simulink model "Parents Phone-MS"  (R2023a)
settings: Solver=FixedStepAuto  StartTime=0.0  StopTime=inf  RelTol=1e-3
undefined symbols (not defined in the file): alti, latitude_, Longit, udp_recieve0x2810x29
libraries: androidcommunicationlib x5, androiduilib x3, androidaudiovideolib x1
settings Model: Creator=91942  LastModifiedBy=ketha
settings OptimizationCC: EnhancedBackFolding=on  PassReuseOutputArgsAs=Individual arguments  ZeroExternalMemoryAtStartup=off  ZeroInternalMemoryAtStartup=off  MaxStackSize=64  OptimizeBlockOrder=speed  DifferentSizesBufferReuse=on  OptimizationCustomize=off  EfficientTunableParamExpr=on
settings DebuggingCC: ParameterTunabilityLossMsg=error
settings HardwareCC: ProdBitPerLong=64  ProdLargestAtomicInteger=LongLong  ProdLargestAtomicFloat=Double  ProdLongLongMode=on  ProdHWDeviceType=ARM Compatible->ARM 64-bit (LP64)  UseEmbeddedCoderFeatures=off
settings SFSimCC: MATLABDynamicMemAlloc=off
settings RTWCC: Description=Embedded Coder  SystemTargetFile=ert.tlc  HardwareBoard=Android Device (64bit)  TLCOptions="-aInlineSetEventsForThisBaseRateFcn=TLC_FALSE -aSuppressMultiTaskScheduler=TLC_FALSE  -aRateBasedStepFcn=0"  TemplateMakefile=ert_default_tmf  RTWVerbose=off  Toolchain=Android SDK/NDK Tools
settings CodeAppCC: ForceParamTrailComments=on  IgnoreCustomStorageClasses=off  OperatorAnnotations=on  SimulinkDataObjDesc=on  SFDataObjDesc=on  InsertBlockDesc=on
settings ERTTargetCC: SupportNonInlinedSFcns=on

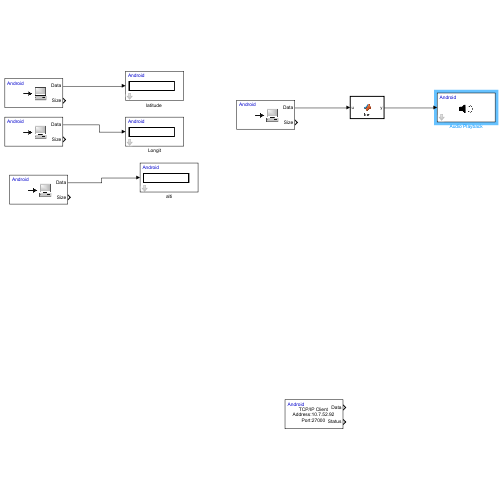
[thumbnail: Simulink's stored preview of the top-level diagram]
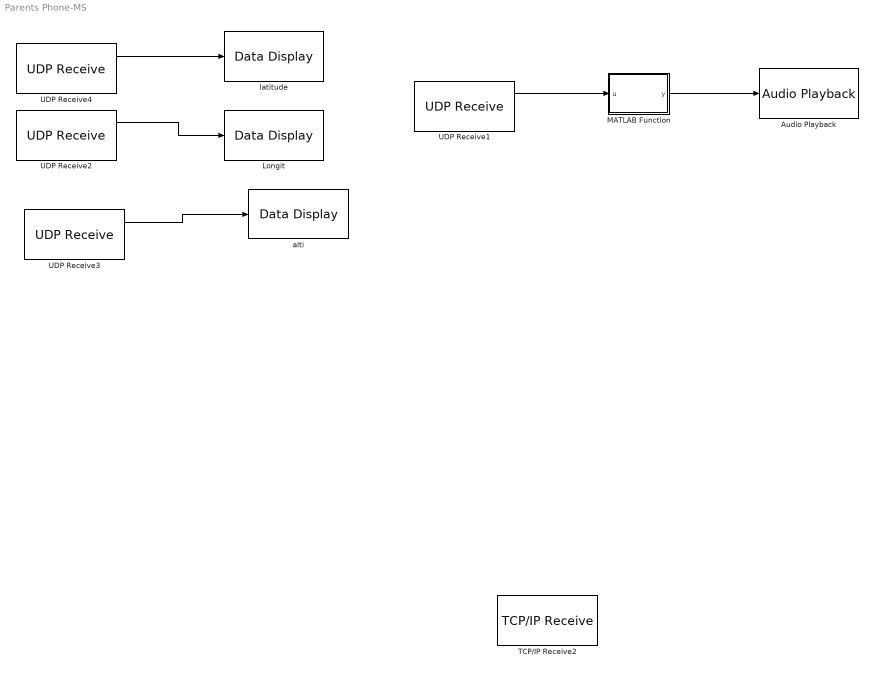
== system Parents Phone-MS ==
  Audio Playback : androidaudiovideolib/Audio Playback  SampleFreq=44100  AudioSamplingFreq=44100  SampleTime=0.1  DeviceStr=0  QueueDuration=0  BlockPlatform=Android
  Longit : androiduilib/Data Display  DataDisplayId=udp_recieve0x2810x29/Longit  Format=Float  Precision=6  SimulateUsing=Code generation  blockPlatform=Android
  MATLAB Function : MATLAB Function  TreatAsAtomicUnit=on
  TCP/IP Receive2 : androidcommunicationlib/TCP//IP Receive  TCPReceiveId=udp_recieve0x2810x29/TCP//IP_Receive2  Mode_=Client  LocalServerPort_=27000  RemoteAddr_=10.7.52.92  RemoteServerPort_=27000  DataType_=uint8  DataSize_=1  SampleTime_=0.1  ClientPortBindingSelection_=off  ClientPortToBind_=35000  BlockingMode_=off  BlockTimeout_=0.1
  UDP Receive1 : androidcommunicationlib/UDP Receive  localURL='0.0.0.0'  localPort=32000  remoteURL='0.0.0.0'  remotePort=-1  recvBufferSize=8192  signalDatatype=int16  dims=8820  isVarSize=off  showBlockingTime=off  blockingTime=0  sampletime=0.1  blockPlatform=Android
  UDP Receive2 : androidcommunicationlib/UDP Receive  localURL='0.0.0.0'  localPort=26000  remoteURL='0.0.0.0'  remotePort=-1  recvBufferSize=8192  signalDatatype=double  dims=1  isVarSize=off  showBlockingTime=off  blockingTime=0  sampletime=0.1  blockPlatform=Android
  UDP Receive3 : androidcommunicationlib/UDP Receive  localURL='0.0.0.0'  localPort=27000  remoteURL='0.0.0.0'  remotePort=-1  recvBufferSize=8192  signalDatatype=double  dims=1  isVarSize=off  showBlockingTime=off  blockingTime=0  sampletime=0.1  blockPlatform=Android
  UDP Receive4 : androidcommunicationlib/UDP Receive  localURL='0.0.0.0'  localPort=25000  remoteURL='0.0.0.0'  remotePort=-1  recvBufferSize=8192  signalDatatype=double  dims=1  isVarSize=off  showBlockingTime=off  blockingTime=0  sampletime=0.1  blockPlatform=Android
  alti : androiduilib/Data Display  DataDisplayId=udp_recieve0x2810x29/alti  Format=Float  Precision=6  SimulateUsing=Code generation  blockPlatform=Android
  "latitude " : androiduilib/Data Display  DataDisplayId=udp_recieve0x2810x29/latitude_  Format=Float  Precision=6  SimulateUsing=Code generation  blockPlatform=Android
  wires:
  UDP Receive1/1 -> MATLAB Function/1(u)
  MATLAB Function/1(y) -> Audio Playback/1
  UDP Receive4/1 -> "latitude "/1
  UDP Receive2/1 -> Longit/1
  UDP Receive3/1 -> alti/1

== matlab function Parents Phone-MS/MATLAB Function ==
  data: u input; y output
function y = fcn(u)
n = length(u) / 2; % Calculate the value of n
z = reshape(u, [n, 2]);

% Convert to int16
y = int16(z);
